simulink model "psbpwm"  (Simulink 6.0)
settings: Solver=ode23tb  SolverMode=SingleTasking  StartTime=0.0  StopTime=1  MaxStep=10e-6  RelTol=1e-4
InitFcn:
  | powericon('psbinitsys',bdroot);
libraries: powerlib2 x7, powerlib_extras x1
settings Model: Creator=patrice  LastModifiedBy=batserve  ExtModeTrigMode=oneshot  ExtModeArmWhenConnect=off  ExtModeAutoUpdateStatusClock=off
settings DataIOCC: ExternalInput=[]  LimitDataPoints=off  SaveOutput=off  TimeSaveName=t  SignalLoggingName=sigsOut
settings OptimizationCC: BlockReduction=off  BooleanDataType=off
settings DebuggingCC: CheckExecutionContextPreStartOutputMsg=on  CheckExecutionContextRuntimeOutputMsg=on  SolverPrmCheckMsg=none  UnconnectedInputMsg=none  UnconnectedOutputMsg=none
settings HardwareCC: TargetUnknown=on
settings RTWCC: TemplateMakefile=grt_unix.tmf

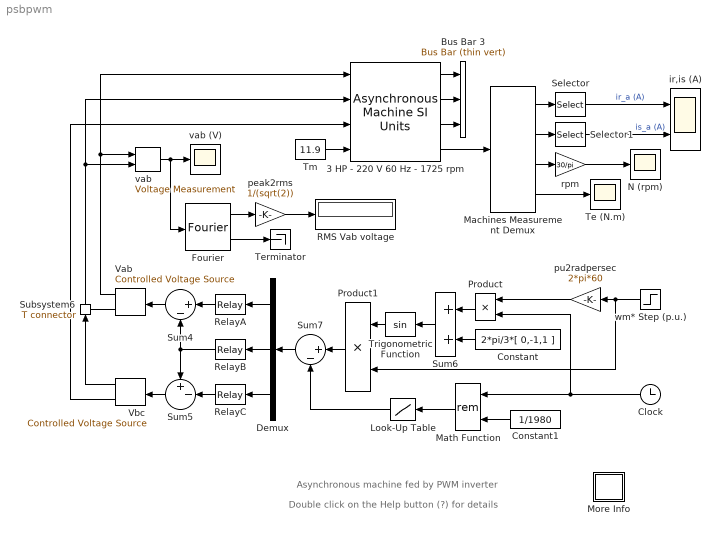
== system psbpwm ==
  note: Asynchronous machine fed by PWM inverter
  note: Double click on the Help button (?) for details
  3 HP - 220 V 60 Hz - 1725 rpm : powerlib2/Machines/Asynchronous Machine SI Units  Tag=PoWeRsYsTeMbLoCk  rotType=Wound  ctrl=Stationary  x1=[ 3*746, 220, 60 ]  x2="[ 0.435  2*2.0e-3 ]"  x3="[ 0.816  2.0e-3 ]"  x4=69.31e-3  x5="[ 0.089  0  2 ]"  x6="[ 1,0   0,0,0   0,0,0 ]"  PSBOutputType=1110  iounits=1  LoadFlowParameters=0
  Bus Bar 3 : powerlib2/Connectors/Bus Bar (thin vert)  input=3  output=0  PSBOutputType=111111111111111111111111111111111111111111111111111111111111111111111111111111111111
  Clock : Clock
      settings: Decimation=10
  Constant : Constant  Orientation=left  Value=2*pi/3*[ 0,-1,1 ]
  Constant1 : Constant  Orientation=left  Value=1/1980
  Demux : Demux  Orientation=left  Outputs=3
  Fourier : powerlib_extras/Measurements/Fourier  f1=60  n=1
  Look-Up Table : Lookup  Orientation=left  DialogController=Simulink.DDGSource  InputValues="[0 0.25  0.75  1] / 1980"  OutputValues="[0  1  -1  0]"  SaturateOnIntegerOverflow=on
  Machines Measurement Demux : powerlib2/Machines/Machines Measurement Demux  machType=Asynchronous  ssm1=on  ssm2=on  ssm3=on  ssm4=on  ssm5=on  ssm6=on  sm1=on  sm2=on  sm3=on  sm4=on  sm5=on  sm6=on  sm7=on  sm8=on  sm9=on  sm10=on  sm11=on  sm115=off  sm12=off  sm13=off  sm14=off  asm1=on  asm2=off  asm3=off  asm4=off  asm5=on  asm6=off  asm7=off  asm8=off  asm9=on  asm10=on  asm11=off  pmsm1=on  pmsm2=on  pmsm3=on  pmsm4=on  pmsm5=on  pmsm6=on  lastType=3
  Math Function : Math  Orientation=left  Operator=rem  SaturateOnIntegerOverflow=on
  More Info : Subsystem
      mask Display: disp('?')
  N (rpm) : Scope
      settings: TimeRange=1  YMin=-200  YMax=1800  DataFormat=Structure
  Product : Product  Orientation=left  SaturateOnIntegerOverflow=on  InputSameDT=on
  Product1 : Product  Orientation=left  SaturateOnIntegerOverflow=on  InputSameDT=on
  RMS Vab voltage : Display
      settings: Decimation=100
  RelayA : Relay  Orientation=left  OnSwitchValue=0  OffSwitchValue=0  OnOutputValue=220*sqrt(2/3)  OffOutputValue=-220*sqrt(2/3)
  RelayB : Relay  Orientation=left  OnSwitchValue=0  OffSwitchValue=0  OnOutputValue=220*sqrt(2/3)  OffOutputValue=-220*sqrt(2/3)
  RelayC : Relay  Orientation=left  OnSwitchValue=0  OffSwitchValue=0  OnOutputValue=220*sqrt(2/3)  OffOutputValue=-220*sqrt(2/3)
  Selector : Selector  InputPortWidth=3
  Selector1 : Selector  InputPortWidth=3
  Subsystem6 : powerlib2/Connectors/T connector  Tag=PoWeRsYsTeMbLoCk  Orientation=up  PSBOutputType=1
  Sum4 : Sum  Orientation=left  Inputs=|+-  SaturateOnIntegerOverflow=on  InputSameDT=on
  Sum5 : Sum  Orientation=left  Inputs=+-|  SaturateOnIntegerOverflow=on  InputSameDT=on
  Sum6 : Sum  Orientation=left  SaturateOnIntegerOverflow=on  InputSameDT=on
  Sum7 : Sum  Orientation=left  Inputs=|+-  SaturateOnIntegerOverflow=on  InputSameDT=on
  Te (N.m) : Scope
      settings: YMin=-30  YMax=100  DataFormat=Structure
  Terminator : Terminator
  Tm : Constant  Value=11.9
  Trigonometric Function : Trigonometry  Orientation=left
  Vab : powerlib2/Electrical Sources/Controlled Voltage Source  Tag=PoWeRsYsTeMbLoCk  Orientation=left  initsrc=on  srctyp=AC  iv=0  iph=0  ifreq=0  mesure=None  PSBOutputType=11
  Vbc : powerlib2/Electrical Sources/Controlled Voltage Source  Tag=PoWeRsYsTeMbLoCk  Orientation=left  initsrc=on  srctyp=AC  iv=0  iph=0  ifreq=0  mesure=None  PSBOutputType=11
  ir,is (A) : Scope  NumInputPorts=2
      settings: YMin=-90~-90  YMax=90~90  DataFormat=Structure
  peak2rms : Gain  Gain=1/(sqrt(2))  SaturateOnIntegerOverflow=on
  pu2radpersec : Gain  Orientation=left  Gain=2*pi*60  SaturateOnIntegerOverflow=on
  rpm : Gain  Gain=30/pi  SaturateOnIntegerOverflow=on
  vab : powerlib2/Measurements/Voltage Measurement  Tag=PoWeRsYsTeMmEaSuReMeNt  PhasorSimulation=off  OutputType=Magnitude  PSBOutputType=0  PSBequivalent=0
  vab (V) : Scope
      settings: TimeRange=0.1  YMin=-400  YMax=400  DataFormat=Structure
  wm* Step (p.u.) : Step  Orientation=left  Time=0  SampleTime=0
  wires:
  Tm/1 -> 3 HP - 220 V 60 Hz - 1725 rpm/4
  3 HP - 220 V 60 Hz - 1725 rpm/4 -> Machines Measurement Demux/1
  Sum4/1 -> Vab/1
  Sum5/1 -> Vbc/1
  Vbc/2 -> 3 HP - 220 V 60 Hz - 1725 rpm/3
  Vab/2 -> Subsystem6/Enable
  Vbc/1 -> Subsystem6/1
  RelayA/1 -> Sum4/1
  RelayC/1 -> Sum5/2
  RelayB/1 -> Sum5/1, Sum4/2
  Demux/2 -> RelayB/1
  Demux/3 -> RelayC/1
  Demux/1 -> RelayA/1
  Sum7/1 -> Demux/1
  pu2radpersec/1 -> Product/1
  Sum6/1 -> Trigonometric Function/1
  Trigonometric Function/1 -> Product1/1
  Product1/1 -> Sum7/1
  wm* Step (p.u.)/1 -> pu2radpersec/1, Product1/2
  Look-Up Table/1 -> Sum7/2
  Clock/1 -> Product/2, Math Function/1
  Math Function/1 -> Look-Up Table/1
  Constant1/1 -> Math Function/2
  Product/1 -> Sum6/1
  Constant/1 -> Sum6/2
  Vab/1 -> 3 HP - 220 V 60 Hz - 1725 rpm/1, vab/1
  Subsystem6/1 -> 3 HP - 220 V 60 Hz - 1725 rpm/2, vab/2
  vab/1 -> vab (V)/1, Fourier/1
  Fourier/1 -> peak2rms/1
  peak2rms/1 -> RMS Vab voltage/1
  Fourier/2 -> Terminator/1
  Machines Measurement Demux/1 -> Selector/1
  Machines Measurement Demux/3 -> rpm/1
  Machines Measurement Demux/4 -> Te (N.m)/1
  Machines Measurement Demux/2 -> Selector1/1
  3 HP - 220 V 60 Hz - 1725 rpm/3 -> Bus Bar 3/3
  3 HP - 220 V 60 Hz - 1725 rpm/2 -> Bus Bar 3/2
  3 HP - 220 V 60 Hz - 1725 rpm/1 -> Bus Bar 3/1
  Selector/1 -> ir,is (A)/1  "ir_a (A)"
  Selector1/1 -> ir,is (A)/2  "is_a (A)"
  rpm/1 -> N (rpm)/1

== system psbpwm/More Info ==
  note: Demonstration
  note: Circuit Description
  note: This demonstration illustrates use of the asynchronous machine
      | in an open-loop speed control on a 3 HP 220 V industrial motor
  note: A three-phase motor rated 3 HP, 220 V, 1725 rpm is fed by a sinusoidal PWM inverter. The base frequency
      | of the sinusoidal reference wave is 60 Hz while the triangular carrier wave's frequency is set to 1980 Hz.
      | The PWM inverter is built entirely with standard Simulink blocks. Its output goes through Controlled Voltage
      | Source blocks before being applied to the Asynchronous Machine block's stator windings. The machine's
      | rotor is short-circuited. Its stator leakage inductance Lls is set to twice its actual value to simulate the
      | effect of a smoothing reactor placed between the inverter and the machine. The load torque applied to the
      | machine's shaft is constant and set to its nominal value of 11.9 N.m.
      |
      | The motor is started from stall. The speed setpoint is set to 1.0 pu, or 1725 rpm. This speed is reached
      | after 0.9 s.
  note: Take a look at the simulation parameters. The Maximum time step has been limited to 10 microseconds.
      | This is required due to the relatively high switching frequency (1980 Hz) of the inverter.
      |
      | Observe that the rotor and stator currents are quite "noisy", despite the use of a smoothing reactor. The noise
      | introduced by the PWM inverter is also observed in the electromagnetic torque waveform Te. However, the
      | motor's inertia prevents this noise from appearing in the motor's speed waveform.
      |
      | The rms value of the fundamental component of the line voltage at the machine's stator terminals is extracted
      | with a Fourier block, which can be found in the Measurements group of the Extras library.
      |
      | Finally, observe the PWM inverter's output. Use the zoom on the vab oscilloscope to zoom in on the waveform.
  note: Louis-A. Dessaint and R. Champagne (Ecole de Technologie Superieure, Montreal)
